simulink model "velocity_integrator"  (R2023b)
settings: Solver=ode15s  StartTime=0.0  StopTime=1  RelTol=1e-3
undefined symbols (not defined in the file): K, Ki
settings Model: PacingRate=1000  Creator=Beniamino  LastModifiedBy=Beniamino

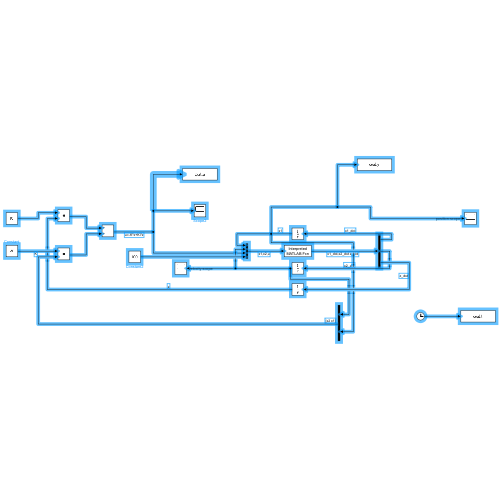
[thumbnail: Simulink's stored preview of the top-level diagram]
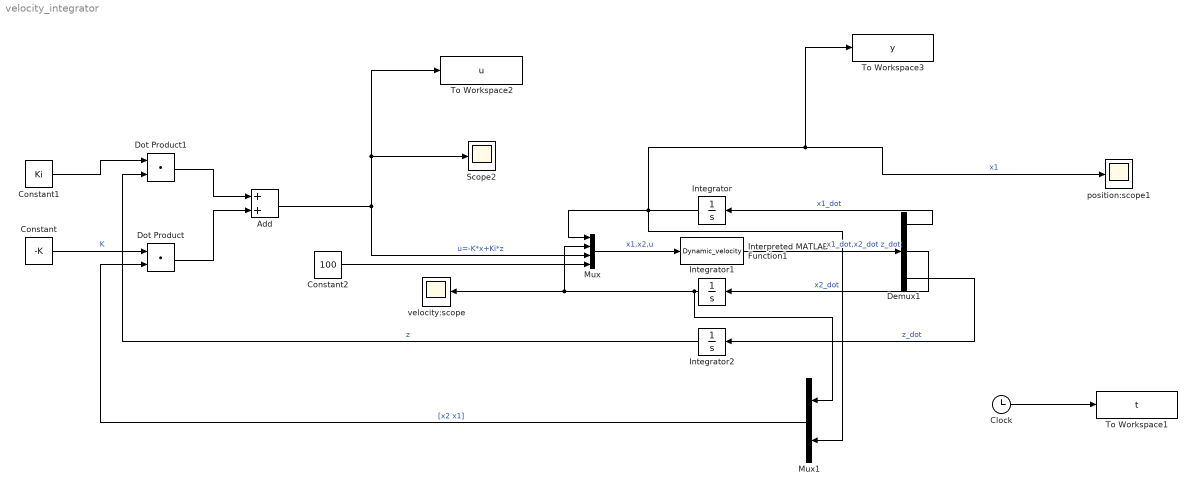
== system velocity_integrator ==
  Add : Sum
  Clock : Clock
  Constant : Constant  Value=-K
  Constant1 : Constant  Value=Ki
  Constant2 : Constant  Value=100
  Demux1 : Demux  Outputs=3
  Dot Product : DotProduct  OutDataTypeStr=Inherit: Inherit via internal rule
  Dot Product1 : DotProduct  OutDataTypeStr=Inherit: Inherit via internal rule
  Integrator : Integrator
  Integrator1 : Integrator
  Integrator2 : Integrator
  Interpreted MATLAB Function1 : MATLABFcn  MATLABFcn=Dynamic_velocity  OutputDimensions=3  Output1D=off
  Mux : Mux
  Mux1 : Mux  Inputs=2
  Scope2 : Scope
  To Workspace1 : ToWorkspace  VariableName=t  SampleTime=-1
  To Workspace2 : ToWorkspace  VariableName=u  SampleTime=-1
  To Workspace3 : ToWorkspace  VariableName=y  SampleTime=-1
  position:scope1 : Scope
  velocity:scope : Scope
  wires:
  Constant2/1 -> Mux/4
  Add/1 -> To Workspace2/1, Scope2/1, Mux/3  "u=-K*x+Ki*z"
  Integrator2/1 -> Dot Product1/2  "z"
  Demux1/2 -> Integrator1/1  "x2_dot"
  Dot Product/1 -> Add/2
  Dot Product1/1 -> Add/1
  Constant1/1 -> Dot Product1/1
  Clock/1 -> To Workspace1/1
  Integrator1/1 -> Mux1/1, Mux/2, velocity:scope/1
  Demux1/3 -> Integrator2/1  "z_dot"
  Interpreted MATLAB Function1/1 -> Demux1/1  "x1_dot,x2_dot z_dot"
  Mux/1 -> Interpreted MATLAB Function1/1  "x1,x2,u"
  Integrator/1 -> Mux1/2, position:scope1/1, To Workspace3/1, Mux/1  "x1"
  Demux1/1 -> Integrator/1  "x1_dot"
  Constant/1 -> Dot Product/1  "K"
  Mux1/1 -> Dot Product/2  "[x2 x1]"
